simulink model "Adaptive_constant"  (R2018b)
settings: Solver=VariableStepAuto  StartTime=0.0  StopTime=60  RelTol=1e-3
libraries: Solver_SF x1, simulink x1
settings Model: Creator=周迅  LastModifiedBy=Administrator

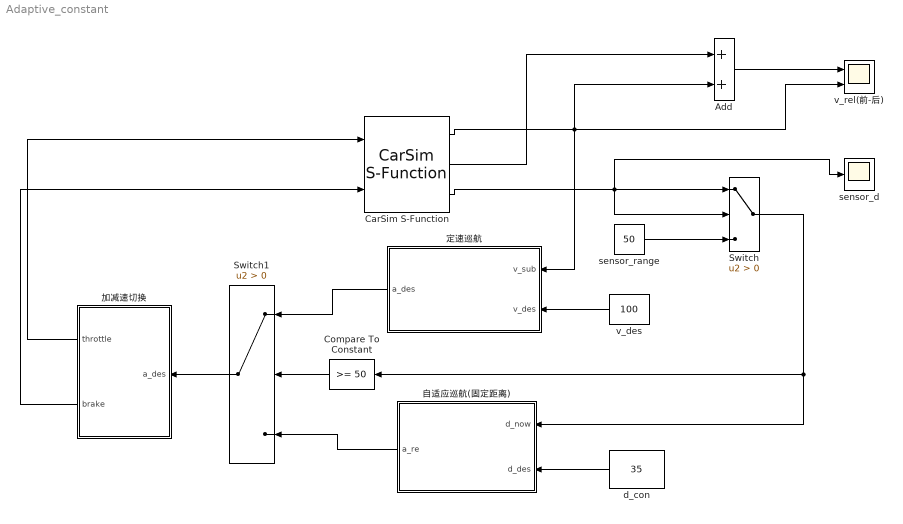
== system Adaptive_constant ==
  Add : Sum
  CarSim S-Function : Solver_SF/CarSim S-Function  Priority=1  SIMFILE=simfile.sim
  Compare To Constant : simulink/Logic and Bit Operations/Compare To Constant  relop=>=  const=50  OutDataTypeStr=boolean
  Switch : Switch  Criteria=u2 > Threshold
  Switch1 : Switch  Criteria=u2 > Threshold
  d_con : Constant  Value=35
  sensor_d : Scope
  sensor_range : Constant  Value=50
  v_des : Constant  Value=100
  v_rel(前-后) : Scope  NumInputPorts=2
  加减速切换 : Subsystem
  定速巡航 : Subsystem
  自适应巡航(固定距离) : Subsystem
  wires:
  Compare To Constant/1 -> Switch1/2
  d_con/1 -> 自适应巡航(固定距离)/2(d_des)
  自适应巡航(固定距离)/1(a_re) -> Switch1/3
  v_des/1 -> 定速巡航/2(v_des)
  CarSim S-Function/3 -> Switch/1, Switch/2, sensor_d/1
  定速巡航/1(a_des) -> Switch1/1
  CarSim S-Function/1 -> v_rel(前-后)/2, Add/2, 定速巡航/1(v_sub)
  CarSim S-Function/2 -> Add/1
  Add/1 -> v_rel(前-后)/1
  Switch1/1 -> 加减速切换/1(a_des)
  加减速切换/1(throttle) -> CarSim S-Function/1
  加减速切换/2(brake) -> CarSim S-Function/2
  sensor_range/1 -> Switch/3
  Switch/1 -> Compare To Constant/1, 自适应巡航(固定距离)/1(d_now)

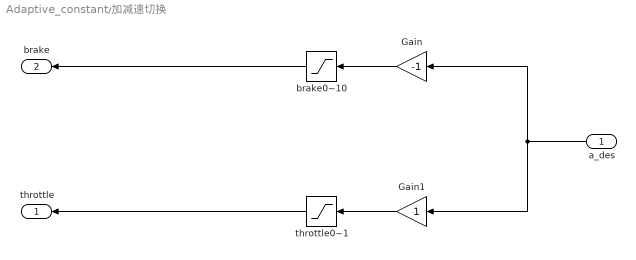
== system Adaptive_constant/加减速切换 ==
  a_des : Inport
  Gain : Gain  Gain=-1
  Gain1 : Gain
  brake0~10 : Saturate  UpperLimit=10  LowerLimit=0
  throttle0~1 : Saturate  UpperLimit=1  LowerLimit=0
  throttle : Outport
  brake : Outport  Port=2
  wires:
  a_des/1 -> Gain/1, Gain1/1
  Gain1/1 -> throttle0~1/1
  Gain/1 -> brake0~10/1
  throttle0~1/1 -> throttle/1
  brake0~10/1 -> brake/1

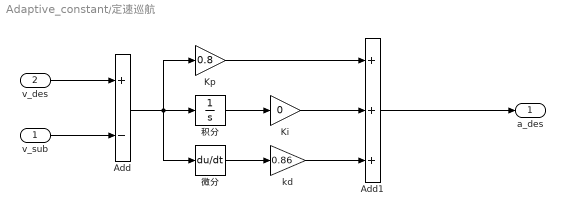
== system Adaptive_constant/定速巡航 ==
  v_sub : Inport
  v_des : Inport  Port=2
  Add : Sum  Inputs=+-
  Add1 : Sum  Inputs=+++
  Ki : Gain  Gain=0
  Kp : Gain  Gain=0.8
  kd : Gain  Gain=0.86
  微分 : Derivative
  积分 : Integrator
  a_des : Outport
  wires:
  Add/1 -> 积分/1, 微分/1, Kp/1
  积分/1 -> Ki/1
  Ki/1 -> Add1/2
  微分/1 -> kd/1
  kd/1 -> Add1/3
  Kp/1 -> Add1/1
  Add1/1 -> a_des/1
  v_des/1 -> Add/1
  v_sub/1 -> Add/2

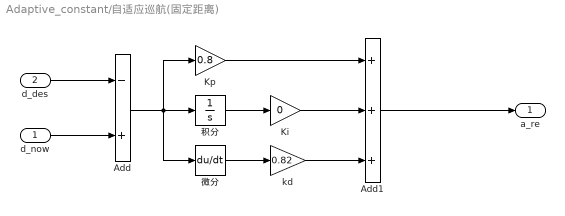
== system Adaptive_constant/自适应巡航(固定距离) ==
  d_now : Inport
  d_des : Inport  Port=2
  Add : Sum  Inputs=-+
  Add1 : Sum  Inputs=+++
  Ki : Gain  Gain=0
  Kp : Gain  Gain=0.8
  kd : Gain  Gain=0.82
  微分 : Derivative
  积分 : Integrator
  a_re : Outport
  wires:
  Add/1 -> 积分/1, 微分/1, Kp/1
  积分/1 -> Ki/1
  Ki/1 -> Add1/2
  微分/1 -> kd/1
  kd/1 -> Add1/3
  Kp/1 -> Add1/1
  Add1/1 -> a_re/1
  d_des/1 -> Add/1
  d_now/1 -> Add/2
